simulink model "Copy_of_Heat_exchanger_model"  (R2016a)
settings: Solver=VariableStepAuto  StartTime=0.0  StopTime=450  FixedStep=0.0001  RelTol=1e-3  AbsTol=1e-3
libraries: simulink x1
settings Model: Creator=EBUKA  LastModifiedBy=EBUKA
settings SolverCC: AlgebraicLoopSolver=LineSearch
settings GRTTargetCC: GeneratePreprocessorConditionals=Use local settings
settings SimscapeCC: SimscapeLogType=all  SimscapeLogDataHistory=10000

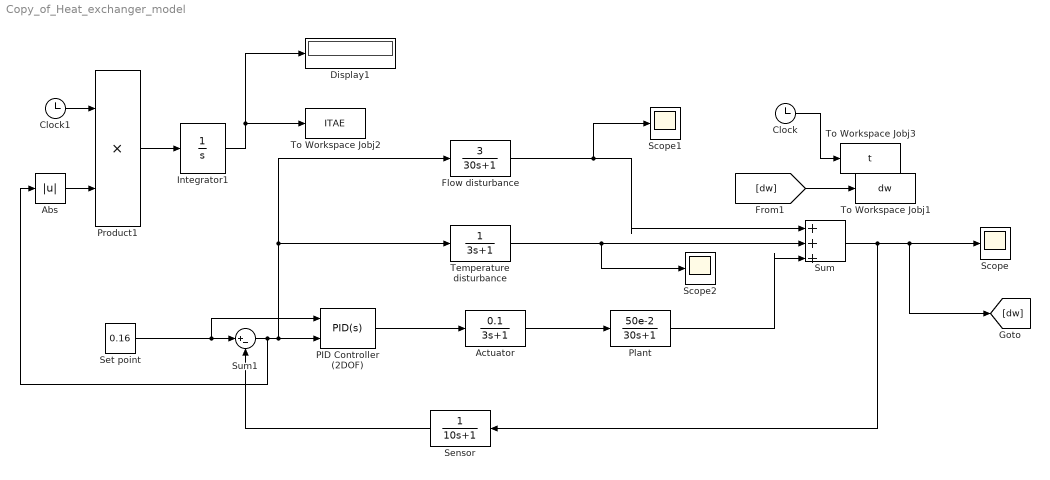
== system Copy_of_Heat_exchanger_model ==
  Abs : Abs
  Actuator : TransferFcn  Numerator=[0.1]  Denominator=[3 1]
  Clock : Clock
  Clock1 : Clock
  Display1 : Display
  Flow disturbance : TransferFcn  Numerator=[3]  Denominator=[30 1]
  Integrator1 : Integrator
  PID Controller (2DOF) : simulink/Continuous/PID Controller (2DOF)  Controller=PID  TimeDomain=Continuous-time  SampleTime=-1  IntegratorMethod=Forward Euler  FilterMethod=Forward Euler  Form=Parallel  UseFilter=on  ControllerParametersSource=internal  P=-213.074808445691  I=-16.5495338320983  D=-656.890310322411  N=17.7832505479324  b=0.0142668624506504  c=9.77482946575499e-05  InitialConditionSource=internal  InitialConditionForIntegrator=0  InitialConditionForFilter=0  ExternalReset=none  LimitOutput=off  UpperSaturationLimit=inf  LowerSaturationLimit=-inf  LinearizeAsGain=on  AntiWindupMode=none  Kb=1  TrackingMode=off  Kt=1  PParamMin=[]  PParamMax=[]  IParamMin=[]  IParamMax=[]  DParamMin=[]  DParamMax=[]  NParamMin=[]  NParamMax=[]  bParamMin=[]  bParamMax=[]  cParamMin=[]  cParamMax=[]  KbParamMin=[]  KbParamMax=[]  KtParamMin=[]  KtParamMax=[]  POutMin=[]  POutMax=[]  IOutMin=[]  IOutMax=[]  DOutMin=[]  DOutMax=[]  NOutMin=[]  NOutMax=[]  bOutMin=[]  bOutMax=[]  cOutMin=[]  cOutMax=[]  KbOutMin=[]  KbOutMax=[]  KtOutMin=[]  KtOutMax=[]  IntegratorOutMin=[]  IntegratorOutMax=[]  FilterOutMin=[]  FilterOutMax=[]  SumOutMin=[]  SumOutMax=[]  Sum1OutMin=[]  Sum1OutMax=[]  Sum2OutMin=[]  Sum2OutMax=[]  Sum3OutMin=[]  Sum3OutMax=[]  SumI1OutMin=[]  SumI1OutMax=[]  SumI2OutMin=[]  SumI2OutMax=[]  SumI3OutMin=[]  SumI3OutMax=[]  SumDOutMin=[]  SumDOutMax=[]  SaturationOutMin=[]  SaturationOutMax=[]  IntegratorContinuousStateAttributes=''  IntegratorStateMustResolveToSignalObject=off  IntegratorRTWStateStorageClass=Auto  FilterContinuousStateAttributes=''  FilterStateMustResolveToSignalObject=off  FilterRTWStateStorageClass=Auto  DifferentiatorICPrevScaledInput=0  DifferentiatorOutMin=[]  DifferentiatorOutMax=[]
  Plant : TransferFcn  Numerator=[50e-2]  Denominator=[30 1]
  Product1 : Product
  Scope : Scope
  Scope1 : Scope
  Scope2 : Scope
  Sensor : TransferFcn  Denominator=[10 1]
  Set point : Constant  Value=0.16
  Sum : Sum  Inputs=|+|+|+
  Sum1 : Sum  Inputs=|+-
  Temperature disturbance : TransferFcn  Denominator=[3 1]
  To Workspace Jobj1 : ToWorkspace  VariableName=dw  SampleTime=-1
  To Workspace Jobj2 : ToWorkspace  VariableName=ITAE  SampleTime=-1
  To Workspace Jobj3 : ToWorkspace  VariableName=t  SampleTime=-1
  wires:
  Temperature disturbance/1 -> Scope2/1, Sum/2
  Plant/1 -> Sum/3
  Actuator/1 -> Plant/1
  Sensor/1 -> Sum1/2
  Sum/1 -> [dw], Scope/1, Sensor/1
  Clock/1 -> To Workspace Jobj3/1
  [dw] -> To Workspace Jobj1/1
  Flow disturbance/1 -> Scope1/1, Sum/1
  Set point/1 -> PID Controller (2DOF)/1, Sum1/1
  PID Controller (2DOF)/1 -> Actuator/1
  Abs/1 -> Product1/2
  Sum1/1 -> Abs/1, PID Controller (2DOF)/2, Flow disturbance/1, Temperature disturbance/1
  Integrator1/1 -> To Workspace Jobj2/1, Display1/1
  Clock1/1 -> Product1/1
  Product1/1 -> Integrator1/1
